simulink library "inp"  (R2021b)
settings: Solver=VariableStepAuto  StartTime=0.0  StopTime=10.0  RelTol=1e-3
undefined symbols (not defined in the file): C_TASK_5MS_S, FALSE, KINP_AcoreReadyToSlp_flg_ovrdflg, KINP_AcoreReadyToSlp_flg_ovrdval, KINP_AllowMovThd_OTA_enum_ovrdflg, KINP_AllowMovThd_OTA_enum_ovrdval, KINP_APSAngleTarget_Deg_ovrdflg, KINP_APSAngleTarget_Deg_ovrdval, KINP_APSDecReq_mps2_ovrdflg, KINP_APSDecReq_mps2_ovrdval, KINP_APSDecReqA_flg_ovrdflg, KINP_APSDecReqA_flg_ovrdval, KINP_APSDFLL_cm_ovrdflg, KINP_APSDFLL_cm_ovrdval, KINP_APSDFLR_cm_ovrdflg, KINP_APSDFLR_cm_ovrdval, KINP_APSDRLL_cm_ovrdflg, KINP_APSDRLL_cm_ovrdval, KINP_APSDRLR_cm_ovrdflg, KINP_APSDRLR_cm_ovrdval, KINP_APSExitCondition_enum_ovrdflg, KINP_APSExitCondition_enum_ovrdval, KINP_APSHWVer_enum_ovrdflg, KINP_APSHWVer_enum_ovrdval, KINP_APSProgressPCT_pct_ovrdflg, KINP_APSProgressPCT_pct_ovrdval, KINP_APSReq_enum_ovrdflg, KINP_APSReq_enum_ovrdval, KINP_APSRQDisplay_enum_ovrdflg, KINP_APSRQDisplay_enum_ovrdval, KINP_APSRqEPASCtrl_flg_ovrdflg, KINP_APSRqEPASCtrl_flg_ovrdval, KINP_APSShiftPosnReq_enum_ovrdval, KINP_APSShiftPosnReq_enum_ovrflg, KINP_APSSpeedCMD_kph_ovrdval, KINP_APSSpeedCMD_kph_ovrflg, KINP_APSStaSystem_enum_ovrdflg, KINP_APSStaSystem_enum_ovrdval, KINP_APSSWVer_enum_ovrdflg, KINP_APSSWVer_enum_ovrdval, KINP_APSVMCReqA_flg_ovrdval, KINP_APSVMCReqA_flg_ovrflg, KINP_APSVRqEPASCtrl_flg_ovrdflg, KINP_APSVRqEPASCtrl_flg_ovrdval, KINP_AuxBattVolmV_mV_ovrdflg, KINP_AuxBattVolmV_mV_ovrdval, KINP_CAASSta_enum_ovrdflg, KINP_CAASSta_enum_ovrdval, KINP_CAASVMCReqA_flg_ovrdval, KINP_CAASVMCReqA_flg_ovrflg, KINP_Chime_enum_ovrdflg, KINP_Chime_enum_ovrdval, KINP_ClearDTCcmd_flg_ovrdflg, KINP_ClearDTCcmd_flg_ovrdval, KINP_EvccAplusPwrUpReq_flg_ovrdflg, KINP_EvccAplusPwrUpReq_flg_ovrdval, KINP_LFID_raw_ovrdval, KINP_LFID_raw_ovrflg, KINP_LRID_raw_ovrdval, KINP_MemOffsetAccX_raw16_ovrdflg ... (+118)
libraries: FVT_lib x595, hcu_lib x1
(part 11 of 27)

== system inp/INP/CAN1/SignalCheck/ESC5 ==
  BHAL_outputs : Inport
  inp_CanValid_bus : Inport  Port=2
  BrkSwSta : FVT_lib/inp/can_signal_template  SystemSampleTime=-1  VariantActivationTime=update diagram  Latency=0  AutoFrameSizeCalculation=off
      link override defval: Value=KINP_BrkSwSta_flg_defval
      link override fftdec: Value=KINP_BrkSwSta_flg_fftdec
      link override fftinc: Value=KINP_BrkSwSta_flg_fftinc
      link override fftlim: Value=KINP_BrkSwSta_flg_fftlim
      link override invalid: Value=KINP_BrkSwSta_flg_invalid
      link override ovrdflg: Value=KINP_BrkSwSta_flg_ovrdflg
      link override ovrdval: Value=KINP_BrkSwSta_flg_ovrdval
      link override setvalid: Value=KINP_BrkSwSta_flg_setvalid
      link override srvcflg: Value=KINP_BrkSwSta_flg_srvcflg
      link override srvcval: Value=KINP_BrkSwSta_flg_srvcval
  BrkSwV : FVT_lib/inp/can_signal_template  SystemSampleTime=-1  VariantActivationTime=update diagram  Latency=0  AutoFrameSizeCalculation=off
      link override defval: Value=KINP_BrkSwV_flg_defval
      link override fftdec: Value=KINP_BrkSwV_flg_fftdec
      link override fftinc: Value=KINP_BrkSwV_flg_fftinc
      link override fftlim: Value=KINP_BrkSwV_flg_fftlim
      link override invalid: Value=KINP_BrkSwV_flg_invalid
      link override ovrdflg: Value=KINP_BrkSwV_flg_ovrdflg
      link override ovrdval: Value=KINP_BrkSwV_flg_ovrdval
      link override setvalid: Value=KINP_BrkSwV_flg_setvalid
      link override srvcflg: Value=KINP_BrkSwV_flg_srvcflg
      link override srvcval: Value=KINP_BrkSwV_flg_srvcval
  ESC5CRC8 : FVT_lib/inp/can_signal_template  SystemSampleTime=-1  VariantActivationTime=update diagram  Latency=0  AutoFrameSizeCalculation=off
      link override defval: Value=KINP_ESC5CRC8_enum_defval
      link override fftdec: Value=KINP_ESC5CRC8_enum_fftdec
      link override fftinc: Value=KINP_ESC5CRC8_enum_fftinc
      link override fftlim: Value=KINP_ESC5CRC8_enum_fftlim
      link override invalid: Value=KINP_ESC5CRC8_enum_invalid
      link override ovrdflg: Value=KINP_ESC5CRC8_enum_ovrdflg
      link override ovrdval: Value=KINP_ESC5CRC8_enum_ovrdval
      link override setvalid: Value=KINP_ESC5CRC8_enum_setvalid
      link override srvcflg: Value=KINP_ESC5CRC8_enum_srvcflg
      link override srvcval: Value=KINP_ESC5CRC8_enum_srvcval
  ESC5CSErr : FVT_lib/inp/can_signal_template  SystemSampleTime=-1  VariantActivationTime=update diagram  Latency=0  AutoFrameSizeCalculation=off
      link override defval: Value=KINP_ESC5CSErr_flg_defval
      link override fftdec: Value=KINP_ESC5CSErr_flg_fftdec
      link override fftinc: Value=KINP_ESC5CSErr_flg_fftinc
      link override fftlim: Value=KINP_ESC5CSErr_flg_fftlim
      link override invalid: Value=KINP_ESC5CSErr_flg_invalid
      link override ovrdflg: Value=KINP_ESC5CSErr_flg_ovrdflg
      link override ovrdval: Value=KINP_ESC5CSErr_flg_ovrdval
      link override setvalid: Value=KINP_ESC5CSErr_flg_setvalid
      link override srvcflg: Value=KINP_ESC5CSErr_flg_srvcflg
      link override srvcval: Value=KINP_ESC5CSErr_flg_srvcval
  ESC5RC : FVT_lib/inp/can_signal_template  SystemSampleTime=-1  VariantActivationTime=update diagram  Latency=0  AutoFrameSizeCalculation=off
      link override defval: Value=KINP_ESC5RC_enum_defval
      link override fftdec: Value=KINP_ESC5RC_enum_fftdec
      link override fftinc: Value=KINP_ESC5RC_enum_fftinc
      link override fftlim: Value=KINP_ESC5RC_enum_fftlim
      link override invalid: Value=KINP_ESC5RC_enum_invalid
      link override ovrdflg: Value=KINP_ESC5RC_enum_ovrdflg
      link override ovrdval: Value=KINP_ESC5RC_enum_ovrdval
      link override setvalid: Value=KINP_ESC5RC_enum_setvalid
      link override srvcflg: Value=KINP_ESC5RC_enum_srvcflg
      link override srvcval: Value=KINP_ESC5RC_enum_srvcval
  ESC5RCErr : FVT_lib/inp/can_signal_template  SystemSampleTime=-1  VariantActivationTime=update diagram  Latency=0  AutoFrameSizeCalculation=off
      link override defval: Value=KINP_ESC5RCErr_flg_defval
      link override fftdec: Value=KINP_ESC5RCErr_flg_fftdec
      link override fftinc: Value=KINP_ESC5RCErr_flg_fftinc
      link override fftlim: Value=KINP_ESC5RCErr_flg_fftlim
      link override invalid: Value=KINP_ESC5RCErr_flg_invalid
      link override ovrdflg: Value=KINP_ESC5RCErr_flg_ovrdflg
      link override ovrdval: Value=KINP_ESC5RCErr_flg_ovrdval
      link override setvalid: Value=KINP_ESC5RCErr_flg_setvalid
      link override srvcflg: Value=KINP_ESC5RCErr_flg_srvcflg
      link override srvcval: Value=KINP_ESC5RCErr_flg_srvcval
  LatAccel : FVT_lib/inp/can_signal_template  SystemSampleTime=-1  VariantActivationTime=update diagram  Latency=0  AutoFrameSizeCalculation=off
      link override defval: Value=KINP_LatAccel_Gps_defval
      link override fftdec: Value=KINP_LatAccel_Gps_fftdec
      link override fftinc: Value=KINP_LatAccel_Gps_fftinc
      link override fftlim: Value=KINP_LatAccel_Gps_fftlim
      link override invalid: Value=KINP_LatAccel_Gps_invalid
      link override ovrdflg: Value=KINP_LatAccel_Gps_ovrdflg
      link override ovrdval: Value=KINP_LatAccel_Gps_ovrdval
      link override setvalid: Value=KINP_LatAccel_Gps_setvalid
      link override srvcflg: Value=KINP_LatAccel_Gps_srvcflg
      link override srvcval: Value=KINP_LatAccel_Gps_srvcval
  LatAccelV : FVT_lib/inp/can_signal_template  SystemSampleTime=-1  VariantActivationTime=update diagram  Latency=0  AutoFrameSizeCalculation=off
      link override defval: Value=KINP_LatAccelV_flg_defval
      link override fftdec: Value=KINP_LatAccelV_flg_fftdec
      link override fftinc: Value=KINP_LatAccelV_flg_fftinc
      link override fftlim: Value=KINP_LatAccelV_flg_fftlim
      link override invalid: Value=KINP_LatAccelV_flg_invalid
      link override ovrdflg: Value=KINP_LatAccelV_flg_ovrdflg
      link override ovrdval: Value=KINP_LatAccelV_flg_ovrdval
      link override setvalid: Value=KINP_LatAccelV_flg_setvalid
      link override srvcflg: Value=KINP_LatAccelV_flg_srvcflg
      link override srvcval: Value=KINP_LatAccelV_flg_srvcval
  LongAccel : FVT_lib/inp/can_signal_template  SystemSampleTime=-1  VariantActivationTime=update diagram  Latency=0  AutoFrameSizeCalculation=off
      link override defval: Value=KINP_LongAccel_Gps_defval
      link override fftdec: Value=KINP_LongAccel_Gps_fftdec
      link override fftinc: Value=KINP_LongAccel_Gps_fftinc
      link override fftlim: Value=KINP_LongAccel_Gps_fftlim
      link override invalid: Value=KINP_LongAccel_Gps_invalid
      link override ovrdflg: Value=KINP_LongAccel_Gps_ovrdflg
      link override ovrdval: Value=KINP_LongAccel_Gps_ovrdval
      link override setvalid: Value=KINP_LongAccel_Gps_setvalid
      link override srvcflg: Value=KINP_LongAccel_Gps_srvcflg
      link override srvcval: Value=KINP_LongAccel_Gps_srvcval
  LongAccelV : FVT_lib/inp/can_signal_template  SystemSampleTime=-1  VariantActivationTime=update diagram  Latency=0  AutoFrameSizeCalculation=off
      link override defval: Value=KINP_LongAccelV_flg_defval
      link override fftdec: Value=KINP_LongAccelV_flg_fftdec
      link override fftinc: Value=KINP_LongAccelV_flg_fftinc
      link override fftlim: Value=KINP_LongAccelV_flg_fftlim
      link override invalid: Value=KINP_LongAccelV_flg_invalid
      link override ovrdflg: Value=KINP_LongAccelV_flg_ovrdflg
      link override ovrdval: Value=KINP_LongAccelV_flg_ovrdval
      link override setvalid: Value=KINP_LongAccelV_flg_setvalid
      link override srvcflg: Value=KINP_LongAccelV_flg_srvcflg
      link override srvcval: Value=KINP_LongAccelV_flg_srvcval
  MCPressure : FVT_lib/inp/can_signal_template  SystemSampleTime=-1  VariantActivationTime=update diagram  Latency=0  AutoFrameSizeCalculation=off
      link override defval: Value=KINP_MCPressure_bar_defval
      link override fftdec: Value=KINP_MCPressure_bar_fftdec
      link override fftinc: Value=KINP_MCPressure_bar_fftinc
      link override fftlim: Value=KINP_MCPressure_bar_fftlim
      link override invalid: Value=KINP_MCPressure_bar_invalid
      link override ovrdflg: Value=KINP_MCPressure_bar_ovrdflg
      link override ovrdval: Value=KINP_MCPressure_bar_ovrdval
      link override setvalid: Value=KINP_MCPressure_bar_setvalid
      link override srvcflg: Value=KINP_MCPressure_bar_srvcflg
      link override srvcval: Value=KINP_MCPressure_bar_srvcval
  MCPressureV : FVT_lib/inp/can_signal_template  SystemSampleTime=-1  VariantActivationTime=update diagram  Latency=0  AutoFrameSizeCalculation=off
      link override defval: Value=KINP_MCPressureV_flg_defval
      link override fftdec: Value=KINP_MCPressureV_flg_fftdec
      link override fftinc: Value=KINP_MCPressureV_flg_fftinc
      link override fftlim: Value=KINP_MCPressureV_flg_fftlim
      link override invalid: Value=KINP_MCPressureV_flg_invalid
      link override ovrdflg: Value=KINP_MCPressureV_flg_ovrdflg
      link override ovrdval: Value=KINP_MCPressureV_flg_ovrdval
      link override setvalid: Value=KINP_MCPressureV_flg_setvalid
      link override srvcflg: Value=KINP_MCPressureV_flg_srvcflg
      link override srvcval: Value=KINP_MCPressureV_flg_srvcval
  Terminator_{1..14} (14 alike) : Terminator
  True_VHAL_BrkSwSta_flg : Constant  Value=TRUE  OutDataTypeStr=boolean
  True_VHAL_BrkSwV_flg : Constant  Value=TRUE  OutDataTypeStr=boolean
  True_VHAL_ESC5CRC8_enum : Constant  Value=TRUE  OutDataTypeStr=boolean
  True_VHAL_ESC5CSErr_flg : Constant  Value=TRUE  OutDataTypeStr=boolean
  True_VHAL_ESC5RCErr_flg : Constant  Value=TRUE  OutDataTypeStr=boolean
  True_VHAL_ESC5RC_enum : Constant  Value=TRUE  OutDataTypeStr=boolean
  True_VHAL_LatAccelV_flg : Constant  Value=TRUE  OutDataTypeStr=boolean
  True_VHAL_LatAccel_Gps : Constant  Value=TRUE  OutDataTypeStr=boolean
  True_VHAL_LongAccelV_flg : Constant  Value=TRUE  OutDataTypeStr=boolean
  True_VHAL_LongAccel_Gps : Constant  Value=TRUE  OutDataTypeStr=boolean
  True_VHAL_MCPressureV_flg : Constant  Value=TRUE  OutDataTypeStr=boolean
  True_VHAL_MCPressure_bar : Constant  Value=TRUE  OutDataTypeStr=boolean
  True_VHAL_YawRateV_flg : Constant  Value=TRUE  OutDataTypeStr=boolean
  True_VHAL_YawRate_degps : Constant  Value=TRUE  OutDataTypeStr=boolean
  YawRate : FVT_lib/inp/can_signal_template  SystemSampleTime=-1  VariantActivationTime=update diagram  Latency=0  AutoFrameSizeCalculation=off
      link override defval: Value=KINP_YawRate_degps_defval
      link override fftdec: Value=KINP_YawRate_degps_fftdec
      link override fftinc: Value=KINP_YawRate_degps_fftinc
      link override fftlim: Value=KINP_YawRate_degps_fftlim
      link override invalid: Value=KINP_YawRate_degps_invalid
      link override ovrdflg: Value=KINP_YawRate_degps_ovrdflg
      link override ovrdval: Value=KINP_YawRate_degps_ovrdval
      link override setvalid: Value=KINP_YawRate_degps_setvalid
      link override srvcflg: Value=KINP_YawRate_degps_srvcflg
      link override srvcval: Value=KINP_YawRate_degps_srvcval
  YawRateV : FVT_lib/inp/can_signal_template  SystemSampleTime=-1  VariantActivationTime=update diagram  Latency=0  AutoFrameSizeCalculation=off
      link override defval: Value=KINP_YawRateV_flg_defval
      link override fftdec: Value=KINP_YawRateV_flg_fftdec
      link override fftinc: Value=KINP_YawRateV_flg_fftinc
      link override fftlim: Value=KINP_YawRateV_flg_fftlim
      link override invalid: Value=KINP_YawRateV_flg_invalid
      link override ovrdflg: Value=KINP_YawRateV_flg_ovrdflg
      link override ovrdval: Value=KINP_YawRateV_flg_ovrdval
      link override setvalid: Value=KINP_YawRateV_flg_setvalid
      link override srvcflg: Value=KINP_YawRateV_flg_srvcflg
      link override srvcval: Value=KINP_YawRateV_flg_srvcval
  slr1_{1..14} (14 alike) : BusSelector  OutputSignals=VINP_CANMsgValidESC5_flg
  slr_VHAL_BrkSwSta_flg : BusSelector  OutputSignals=VHAL_BrkSwSta_flg
  slr_VHAL_BrkSwV_flg : BusSelector  OutputSignals=VHAL_BrkSwV_flg
  slr_VHAL_ESC5CRC8_enum : BusSelector  OutputSignals=VHAL_ESC5CRC8_enum
  slr_VHAL_ESC5CSErr_flg : BusSelector  OutputSignals=VHAL_ESC5CSErr_flg
  slr_VHAL_ESC5RCErr_flg : BusSelector  OutputSignals=VHAL_ESC5RCErr_flg
  slr_VHAL_ESC5RC_enum : BusSelector  OutputSignals=VHAL_ESC5RC_enum
  slr_VHAL_LatAccelV_flg : BusSelector  OutputSignals=VHAL_LatAccelV_flg
  slr_VHAL_LatAccel_Gps : BusSelector  OutputSignals=VHAL_LatAccel_Gps
  slr_VHAL_LongAccelV_flg : BusSelector  OutputSignals=VHAL_LongAccelV_flg
  slr_VHAL_LongAccel_Gps : BusSelector  OutputSignals=VHAL_LongAccel_Gps
  slr_VHAL_MCPressureV_flg : BusSelector  OutputSignals=VHAL_MCPressureV_flg
  slr_VHAL_MCPressure_bar : BusSelector  OutputSignals=VHAL_MCPressure_bar
  slr_VHAL_YawRateV_flg : BusSelector  OutputSignals=VHAL_YawRateV_flg
  slr_VHAL_YawRate_degps : BusSelector  OutputSignals=VHAL_YawRate_degps
  VINP_ESC5CSErr_flg : Outport
  VINP_ESC5RCErr_flg : Outport  Port=2
  VINP_BrkSwSta_flg : Outport  Port=3
  VINP_BrkSwV_flg : Outport  Port=4
  VINP_ESC5CRC8_enum : Outport  Port=5
  VINP_ESC5RC_enum : Outport  Port=6
  VINP_LatAccel_Gps : Outport  Port=7
  VINP_LatAccelV_flg : Outport  Port=8
  VINP_LongAccel_Gps : Outport  Port=9
  VINP_LongAccelV_flg : Outport  Port=10
  VINP_MCPressure_bar : Outport  Port=11
  VINP_MCPressureV_flg : Outport  Port=12
  VINP_YawRate_degps : Outport  Port=13
  VINP_YawRateV_flg : Outport  Port=14
  wires:
  BHAL_outputs/1 -> [BHAL_outputs]
  inp_CanValid_bus/1 -> [inp_CanValid_bus]
  [BHAL_outputs] -> slr_VHAL_ESC5CSErr_flg/1
  slr_VHAL_ESC5CSErr_flg/1 -> ESC5CSErr/1  "<VHAL_ESC5CSErr_flg>"
  True_VHAL_ESC5CSErr_flg/1 -> ESC5CSErr/2
  [inp_CanValid_bus] -> slr1_1/1
  slr1_1/1 -> ESC5CSErr/3  "<VINP_CANMsgValidESC5_flg>"
  ESC5CSErr/1 -> VINP_ESC5CSErr_flg/1  "VINP_ESC5CSErr_flg"
  ESC5CSErr/2 -> Terminator_1/1
  [BHAL_outputs] -> slr_VHAL_ESC5RCErr_flg/1
  slr_VHAL_ESC5RCErr_flg/1 -> ESC5RCErr/1  "<VHAL_ESC5RCErr_flg>"
  True_VHAL_ESC5RCErr_flg/1 -> ESC5RCErr/2
  [inp_CanValid_bus] -> slr1_2/1
  slr1_2/1 -> ESC5RCErr/3  "<VINP_CANMsgValidESC5_flg>"
  ESC5RCErr/1 -> VINP_ESC5RCErr_flg/1  "VINP_ESC5RCErr_flg"
  ESC5RCErr/2 -> Terminator_2/1
  [BHAL_outputs] -> slr_VHAL_BrkSwSta_flg/1
  slr_VHAL_BrkSwSta_flg/1 -> BrkSwSta/1  "<VHAL_BrkSwSta_flg>"
  True_VHAL_BrkSwSta_flg/1 -> BrkSwSta/2
  [inp_CanValid_bus] -> slr1_3/1
  slr1_3/1 -> BrkSwSta/3  "<VINP_CANMsgValidESC5_flg>"
  BrkSwSta/1 -> VINP_BrkSwSta_flg/1  "VINP_BrkSwSta_flg"
  BrkSwSta/2 -> Terminator_3/1
  [BHAL_outputs] -> slr_VHAL_BrkSwV_flg/1
  slr_VHAL_BrkSwV_flg/1 -> BrkSwV/1  "<VHAL_BrkSwV_flg>"
  True_VHAL_BrkSwV_flg/1 -> BrkSwV/2
  [inp_CanValid_bus] -> slr1_4/1
  slr1_4/1 -> BrkSwV/3  "<VINP_CANMsgValidESC5_flg>"
  BrkSwV/1 -> VINP_BrkSwV_flg/1  "VINP_BrkSwV_flg"
  BrkSwV/2 -> Terminator_4/1
  [BHAL_outputs] -> slr_VHAL_ESC5CRC8_enum/1
  slr_VHAL_ESC5CRC8_enum/1 -> ESC5CRC8/1  "<VHAL_ESC5CRC8_enum>"
  True_VHAL_ESC5CRC8_enum/1 -> ESC5CRC8/2
  [inp_CanValid_bus] -> slr1_5/1
  slr1_5/1 -> ESC5CRC8/3  "<VINP_CANMsgValidESC5_flg>"
  ESC5CRC8/1 -> VINP_ESC5CRC8_enum/1  "VINP_ESC5CRC8_enum"
  ESC5CRC8/2 -> Terminator_5/1
  [BHAL_outputs] -> slr_VHAL_ESC5RC_enum/1
  slr_VHAL_ESC5RC_enum/1 -> ESC5RC/1  "<VHAL_ESC5RC_enum>"
  True_VHAL_ESC5RC_enum/1 -> ESC5RC/2
  [inp_CanValid_bus] -> slr1_6/1
  slr1_6/1 -> ESC5RC/3  "<VINP_CANMsgValidESC5_flg>"
  ESC5RC/1 -> VINP_ESC5RC_enum/1  "VINP_ESC5RC_enum"
  ESC5RC/2 -> Terminator_6/1
  [BHAL_outputs] -> slr_VHAL_LatAccel_Gps/1
  slr_VHAL_LatAccel_Gps/1 -> LatAccel/1  "<VHAL_LatAccel_Gps>"
  True_VHAL_LatAccel_Gps/1 -> LatAccel/2
  [inp_CanValid_bus] -> slr1_7/1
  slr1_7/1 -> LatAccel/3  "<VINP_CANMsgValidESC5_flg>"
  LatAccel/1 -> VINP_LatAccel_Gps/1  "VINP_LatAccel_Gps"
  LatAccel/2 -> Terminator_7/1
  [BHAL_outputs] -> slr_VHAL_LatAccelV_flg/1
  slr_VHAL_LatAccelV_flg/1 -> LatAccelV/1  "<VHAL_LatAccelV_flg>"
  True_VHAL_LatAccelV_flg/1 -> LatAccelV/2
  [inp_CanValid_bus] -> slr1_8/1
  slr1_8/1 -> LatAccelV/3  "<VINP_CANMsgValidESC5_flg>"
  LatAccelV/1 -> VINP_LatAccelV_flg/1  "VINP_LatAccelV_flg"
  LatAccelV/2 -> Terminator_8/1
  [BHAL_outputs] -> slr_VHAL_LongAccel_Gps/1
  slr_VHAL_LongAccel_Gps/1 -> LongAccel/1  "<VHAL_LongAccel_Gps>"
  True_VHAL_LongAccel_Gps/1 -> LongAccel/2
  [inp_CanValid_bus] -> slr1_9/1
  slr1_9/1 -> LongAccel/3  "<VINP_CANMsgValidESC5_flg>"
  LongAccel/1 -> VINP_LongAccel_Gps/1  "VINP_LongAccel_Gps"
  LongAccel/2 -> Terminator_9/1
  [BHAL_outputs] -> slr_VHAL_LongAccelV_flg/1
  slr_VHAL_LongAccelV_flg/1 -> LongAccelV/1  "<VHAL_LongAccelV_flg>"
  True_VHAL_LongAccelV_flg/1 -> LongAccelV/2
  [inp_CanValid_bus] -> slr1_10/1
  slr1_10/1 -> LongAccelV/3  "<VINP_CANMsgValidESC5_flg>"
  LongAccelV/1 -> VINP_LongAccelV_flg/1  "VINP_LongAccelV_flg"
  LongAccelV/2 -> Terminator_10/1
  [BHAL_outputs] -> slr_VHAL_MCPressure_bar/1
  slr_VHAL_MCPressure_bar/1 -> MCPressure/1  "<VHAL_MCPressure_bar>"
  True_VHAL_MCPressure_bar/1 -> MCPressure/2
  [inp_CanValid_bus] -> slr1_11/1
  slr1_11/1 -> MCPressure/3  "<VINP_CANMsgValidESC5_flg>"
  MCPressure/1 -> VINP_MCPressure_bar/1  "VINP_MCPressure_bar"
  MCPressure/2 -> Terminator_11/1
  [BHAL_outputs] -> slr_VHAL_MCPressureV_flg/1
  slr_VHAL_MCPressureV_flg/1 -> MCPressureV/1  "<VHAL_MCPressureV_flg>"
  True_VHAL_MCPressureV_flg/1 -> MCPressureV/2
  [inp_CanValid_bus] -> slr1_12/1
  slr1_12/1 -> MCPressureV/3  "<VINP_CANMsgValidESC5_flg>"
  MCPressureV/1 -> VINP_MCPressureV_flg/1  "VINP_MCPressureV_flg"
  MCPressureV/2 -> Terminator_12/1
  [BHAL_outputs] -> slr_VHAL_YawRate_degps/1
  slr_VHAL_YawRate_degps/1 -> YawRate/1  "<VHAL_YawRate_degps>"
  True_VHAL_YawRate_degps/1 -> YawRate/2
  [inp_CanValid_bus] -> slr1_13/1
  slr1_13/1 -> YawRate/3  "<VINP_CANMsgValidESC5_flg>"
  YawRate/1 -> VINP_YawRate_degps/1  "VINP_YawRate_degps"
  YawRate/2 -> Terminator_13/1
  [BHAL_outputs] -> slr_VHAL_YawRateV_flg/1
  slr_VHAL_YawRateV_flg/1 -> YawRateV/1  "<VHAL_YawRateV_flg>"
  True_VHAL_YawRateV_flg/1 -> YawRateV/2
  [inp_CanValid_bus] -> slr1_14/1
  slr1_14/1 -> YawRateV/3  "<VINP_CANMsgValidESC5_flg>"
  YawRateV/1 -> VINP_YawRateV_flg/1  "VINP_YawRateV_flg"
  YawRateV/2 -> Terminator_14/1

== system inp/INP/CAN1/SignalCheck/ESC6 ==
  BHAL_outputs : Inport
  inp_CanValid_bus : Inport  Port=2
  ActBrkLampSta : FVT_lib/inp/can_signal_template  SystemSampleTime=-1  VariantActivationTime=update diagram  Latency=0  AutoFrameSizeCalculation=off
      link override defval: Value=KINP_ActBrkLampSta_flg_defval
      link override fftdec: Value=KINP_ActBrkLampSta_flg_fftdec
      link override fftinc: Value=KINP_ActBrkLampSta_flg_fftinc
      link override fftlim: Value=KINP_ActBrkLampSta_flg_fftlim
      link override invalid: Value=KINP_ActBrkLampSta_flg_invalid
      link override ovrdflg: Value=KINP_ActBrkLampSta_flg_ovrdflg
      link override ovrdval: Value=KINP_ActBrkLampSta_flg_ovrdval
      link override setvalid: Value=KINP_ActBrkLampSta_flg_setvalid
      link override srvcflg: Value=KINP_ActBrkLampSta_flg_srvcflg
      link override srvcval: Value=KINP_ActBrkLampSta_flg_srvcval
  ESCADASSta : FVT_lib/inp/can_signal_template  SystemSampleTime=-1  VariantActivationTime=update diagram  Latency=0  AutoFrameSizeCalculation=off
      link override defval: Value=KINP_ESCADASSta_enum_defval
      link override fftdec: Value=KINP_ESCADASSta_enum_fftdec
      link override fftinc: Value=KINP_ESCADASSta_enum_fftinc
      link override fftlim: Value=KINP_ESCADASSta_enum_fftlim
      link override invalid: Value=KINP_ESCADASSta_enum_invalid
      link override ovrdflg: Value=KINP_ESCADASSta_enum_ovrdflg
      link override ovrdval: Value=KINP_ESCADASSta_enum_ovrdval
      link override setvalid: Value=KINP_ESCADASSta_enum_setvalid
      link override srvcflg: Value=KINP_ESCADASSta_enum_srvcflg
      link override srvcval: Value=KINP_ESCADASSta_enum_srvcval
  ESCAPSSta : FVT_lib/inp/can_signal_template  SystemSampleTime=-1  VariantActivationTime=update diagram  Latency=0  AutoFrameSizeCalculation=off
      link override defval: Value=KINP_ESCAPSSta_enum_defval
      link override fftdec: Value=KINP_ESCAPSSta_enum_fftdec
      link override fftinc: Value=KINP_ESCAPSSta_enum_fftinc
      link override fftlim: Value=KINP_ESCAPSSta_enum_fftlim
      link override invalid: Value=KINP_ESCAPSSta_enum_invalid
      link override ovrdflg: Value=KINP_ESCAPSSta_enum_ovrdflg
      link override ovrdval: Value=KINP_ESCAPSSta_enum_ovrdval
      link override setvalid: Value=KINP_ESCAPSSta_enum_setvalid
      link override srvcflg: Value=KINP_ESCAPSSta_enum_srvcflg
      link override srvcval: Value=KINP_ESCAPSSta_enum_srvcval
  ESCStandstill : FVT_lib/inp/can_signal_template  SystemSampleTime=-1  VariantActivationTime=update diagram  Latency=0  AutoFrameSizeCalculation=off
      link override defval: Value=KINP_ESCStandstill_flg_defval
      link override fftdec: Value=KINP_ESCStandstill_flg_fftdec
      link override fftinc: Value=KINP_ESCStandstill_flg_fftinc
      link override fftlim: Value=KINP_ESCStandstill_flg_fftlim
      link override invalid: Value=KINP_ESCStandstill_flg_invalid
      link override ovrdflg: Value=KINP_ESCStandstill_flg_ovrdflg
      link override ovrdval: Value=KINP_ESCStandstill_flg_ovrdval
      link override setvalid: Value=KINP_ESCStandstill_flg_setvalid
      link override srvcflg: Value=KINP_ESCStandstill_flg_srvcflg
      link override srvcval: Value=KINP_ESCStandstill_flg_srvcval
  Terminator_{1..4} (4 alike) : Terminator
  True_VHAL_ActBrkLampSta_flg : Constant  Value=TRUE  OutDataTypeStr=boolean
  True_VHAL_ESCADASSta_enum : Constant  Value=TRUE  OutDataTypeStr=boolean
  True_VHAL_ESCAPSSta_enum : Constant  Value=TRUE  OutDataTypeStr=boolean
  True_VHAL_ESCStandstill_flg : Constant  Value=TRUE  OutDataTypeStr=boolean
  slr1_{1..4} (4 alike) : BusSelector  OutputSignals=VINP_CANMsgValidESC6_flg
  slr_VHAL_ActBrkLampSta_flg : BusSelector  OutputSignals=VHAL_ActBrkLampSta_flg
  slr_VHAL_ESCADASSta_enum : BusSelector  OutputSignals=VHAL_ESCADASSta_enum
  slr_VHAL_ESCAPSSta_enum : BusSelector  OutputSignals=VHAL_ESCAPSSta_enum
  slr_VHAL_ESCStandstill_flg : BusSelector  OutputSignals=VHAL_ESCStandstill_flg
  VINP_ActBrkLampSta_flg : Outport
  VINP_ESCADASSta_enum : Outport  Port=2
  VINP_ESCAPSSta_enum : Outport  Port=3
  VINP_ESCStandstill_flg : Outport  Port=4
  wires:
  BHAL_outputs/1 -> [BHAL_outputs]
  inp_CanValid_bus/1 -> [inp_CanValid_bus]
  [BHAL_outputs] -> slr_VHAL_ActBrkLampSta_flg/1
  slr_VHAL_ActBrkLampSta_flg/1 -> ActBrkLampSta/1  "<VHAL_ActBrkLampSta_flg>"
  True_VHAL_ActBrkLampSta_flg/1 -> ActBrkLampSta/2
  [inp_CanValid_bus] -> slr1_1/1
  slr1_1/1 -> ActBrkLampSta/3  "<VINP_CANMsgValidESC6_flg>"
  ActBrkLampSta/1 -> VINP_ActBrkLampSta_flg/1  "VINP_ActBrkLampSta_flg"
  ActBrkLampSta/2 -> Terminator_1/1
  [BHAL_outputs] -> slr_VHAL_ESCADASSta_enum/1
  slr_VHAL_ESCADASSta_enum/1 -> ESCADASSta/1  "<VHAL_ESCADASSta_enum>"
  True_VHAL_ESCADASSta_enum/1 -> ESCADASSta/2
  [inp_CanValid_bus] -> slr1_2/1
  slr1_2/1 -> ESCADASSta/3  "<VINP_CANMsgValidESC6_flg>"
  ESCADASSta/1 -> VINP_ESCADASSta_enum/1  "VINP_ESCADASSta_enum"
  ESCADASSta/2 -> Terminator_2/1
  [BHAL_outputs] -> slr_VHAL_ESCAPSSta_enum/1
  slr_VHAL_ESCAPSSta_enum/1 -> ESCAPSSta/1  "<VHAL_ESCAPSSta_enum>"
  True_VHAL_ESCAPSSta_enum/1 -> ESCAPSSta/2
  [inp_CanValid_bus] -> slr1_3/1
  slr1_3/1 -> ESCAPSSta/3  "<VINP_CANMsgValidESC6_flg>"
  ESCAPSSta/1 -> VINP_ESCAPSSta_enum/1  "VINP_ESCAPSSta_enum"
  ESCAPSSta/2 -> Terminator_3/1
  [BHAL_outputs] -> slr_VHAL_ESCStandstill_flg/1
  slr_VHAL_ESCStandstill_flg/1 -> ESCStandstill/1  "<VHAL_ESCStandstill_flg>"
  True_VHAL_ESCStandstill_flg/1 -> ESCStandstill/2
  [inp_CanValid_bus] -> slr1_4/1
  slr1_4/1 -> ESCStandstill/3  "<VINP_CANMsgValidESC6_flg>"
  ESCStandstill/1 -> VINP_ESCStandstill_flg/1  "VINP_ESCStandstill_flg"
  ESCStandstill/2 -> Terminator_4/1

== system inp/INP/CAN1/SignalCheck/ESC7 ==
  BHAL_outputs : Inport
  inp_CanValid_bus : Inport  Port=2
  BrkPedalPos : FVT_lib/inp/can_signal_template  SystemSampleTime=-1  VariantActivationTime=update diagram  Latency=0  AutoFrameSizeCalculation=off
      link override defval: Value=KINP_BrkPedalPos_pct_defval
      link override fftdec: Value=KINP_BrkPedalPos_pct_fftdec
      link override fftinc: Value=KINP_BrkPedalPos_pct_fftinc
      link override fftlim: Value=KINP_BrkPedalPos_pct_fftlim
      link override invalid: Value=KINP_BrkPedalPos_pct_invalid
      link override ovrdflg: Value=KINP_BrkPedalPos_pct_ovrdflg
      link override ovrdval: Value=KINP_BrkPedalPos_pct_ovrdval
      link override setvalid: Value=KINP_BrkPedalPos_pct_setvalid
      link override srvcflg: Value=KINP_BrkPedalPos_pct_srvcflg
      link override srvcval: Value=KINP_BrkPedalPos_pct_srvcval
  BrkPedalPosSta : FVT_lib/inp/can_signal_template  SystemSampleTime=-1  VariantActivationTime=update diagram  Latency=0  AutoFrameSizeCalculation=off
      link override defval: Value=KINP_BrkPedalPosSta_flg_defval
      link override fftdec: Value=KINP_BrkPedalPosSta_flg_fftdec
      link override fftinc: Value=KINP_BrkPedalPosSta_flg_fftinc
      link override fftlim: Value=KINP_BrkPedalPosSta_flg_fftlim
      link override invalid: Value=KINP_BrkPedalPosSta_flg_invalid
      link override ovrdflg: Value=KINP_BrkPedalPosSta_flg_ovrdflg
      link override ovrdval: Value=KINP_BrkPedalPosSta_flg_ovrdval
      link override setvalid: Value=KINP_BrkPedalPosSta_flg_setvalid
      link override srvcflg: Value=KINP_BrkPedalPosSta_flg_srvcflg
      link override srvcval: Value=KINP_BrkPedalPosSta_flg_srvcval
  ESC7CS : FVT_lib/inp/can_signal_template  SystemSampleTime=-1  VariantActivationTime=update diagram  Latency=0  AutoFrameSizeCalculation=off
      link override defval: Value=KINP_ESC7CS_enum_defval
      link override fftdec: Value=KINP_ESC7CS_enum_fftdec
      link override fftinc: Value=KINP_ESC7CS_enum_fftinc
      link override fftlim: Value=KINP_ESC7CS_enum_fftlim
      link override invalid: Value=KINP_ESC7CS_enum_invalid
      link override ovrdflg: Value=KINP_ESC7CS_enum_ovrdflg
      link override ovrdval: Value=KINP_ESC7CS_enum_ovrdval
      link override setvalid: Value=KINP_ESC7CS_enum_setvalid
      link override srvcflg: Value=KINP_ESC7CS_enum_srvcflg
      link override srvcval: Value=KINP_ESC7CS_enum_srvcval
  ESC7CSErr : FVT_lib/inp/can_signal_template  SystemSampleTime=-1  VariantActivationTime=update diagram  Latency=0  AutoFrameSizeCalculation=off
      link override defval: Value=KINP_ESC7CSErr_flg_defval
      link override fftdec: Value=KINP_ESC7CSErr_flg_fftdec
      link override fftinc: Value=KINP_ESC7CSErr_flg_fftinc
      link override fftlim: Value=KINP_ESC7CSErr_flg_fftlim
      link override invalid: Value=KINP_ESC7CSErr_flg_invalid
      link override ovrdflg: Value=KINP_ESC7CSErr_flg_ovrdflg
      link override ovrdval: Value=KINP_ESC7CSErr_flg_ovrdval
      link override setvalid: Value=KINP_ESC7CSErr_flg_setvalid
      link override srvcflg: Value=KINP_ESC7CSErr_flg_srvcflg
      link override srvcval: Value=KINP_ESC7CSErr_flg_srvcval
  ESC7RC : FVT_lib/inp/can_signal_template  SystemSampleTime=-1  VariantActivationTime=update diagram  Latency=0  AutoFrameSizeCalculation=off
      link override defval: Value=KINP_ESC7RC_enum_defval
      link override fftdec: Value=KINP_ESC7RC_enum_fftdec
      link override fftinc: Value=KINP_ESC7RC_enum_fftinc
      link override fftlim: Value=KINP_ESC7RC_enum_fftlim
      link override invalid: Value=KINP_ESC7RC_enum_invalid
      link override ovrdflg: Value=KINP_ESC7RC_enum_ovrdflg
      link override ovrdval: Value=KINP_ESC7RC_enum_ovrdval
      link override setvalid: Value=KINP_ESC7RC_enum_setvalid
      link override srvcflg: Value=KINP_ESC7RC_enum_srvcflg
      link override srvcval: Value=KINP_ESC7RC_enum_srvcval
  ESC7RCErr : FVT_lib/inp/can_signal_template  SystemSampleTime=-1  VariantActivationTime=update diagram  Latency=0  AutoFrameSizeCalculation=off
      link override defval: Value=KINP_ESC7RCErr_flg_defval
      link override fftdec: Value=KINP_ESC7RCErr_flg_fftdec
      link override fftinc: Value=KINP_ESC7RCErr_flg_fftinc
      link override fftlim: Value=KINP_ESC7RCErr_flg_fftlim
      link override invalid: Value=KINP_ESC7RCErr_flg_invalid
      link override ovrdflg: Value=KINP_ESC7RCErr_flg_ovrdflg
      link override ovrdval: Value=KINP_ESC7RCErr_flg_ovrdval
      link override setvalid: Value=KINP_ESC7RCErr_flg_setvalid
      link override srvcflg: Value=KINP_ESC7RCErr_flg_srvcflg
      link override srvcval: Value=KINP_ESC7RCErr_flg_srvcval
  FrRBCActive : FVT_lib/inp/can_signal_template  SystemSampleTime=-1  VariantActivationTime=update diagram  Latency=0  AutoFrameSizeCalculation=off
      link override defval: Value=KINP_FrRBCActive_flg_defval
      link override fftdec: Value=KINP_FrRBCActive_flg_fftdec
      link override fftinc: Value=KINP_FrRBCActive_flg_fftinc
      link override fftlim: Value=KINP_FrRBCActive_flg_fftlim
      link override invalid: Value=KINP_FrRBCActive_flg_invalid
      link override ovrdflg: Value=KINP_FrRBCActive_flg_ovrdflg
      link override ovrdval: Value=KINP_FrRBCActive_flg_ovrdval
      link override setvalid: Value=KINP_FrRBCActive_flg_setvalid
      link override srvcflg: Value=KINP_FrRBCActive_flg_srvcflg
      link override srvcval: Value=KINP_FrRBCActive_flg_srvcval
  FrntAxlTrqReqBrk : FVT_lib/inp/can_signal_template  SystemSampleTime=-1  VariantActivationTime=update diagram  Latency=0  AutoFrameSizeCalculation=off
      link override defval: Value=KINP_FrntAxlTrqReqBrk_Nm_defval
      link override fftdec: Value=KINP_FrntAxlTrqReqBrk_Nm_fftdec
      link override fftinc: Value=KINP_FrntAxlTrqReqBrk_Nm_fftinc
      link override fftlim: Value=KINP_FrntAxlTrqReqBrk_Nm_fftlim
      link override invalid: Value=KINP_FrntAxlTrqReqBrk_Nm_invalid
      link override ovrdflg: Value=KINP_FrntAxlTrqReqBrk_Nm_ovrdflg
      link override ovrdval: Value=KINP_FrntAxlTrqReqBrk_Nm_ovrdval
      link override setvalid: Value=KINP_FrntAxlTrqReqBrk_Nm_setvalid
      link override srvcflg: Value=KINP_FrntAxlTrqReqBrk_Nm_srvcflg
      link override srvcval: Value=KINP_FrntAxlTrqReqBrk_Nm_srvcval
  RDCActive : FVT_lib/inp/can_signal_template  SystemSampleTime=-1  VariantActivationTime=update diagram  Latency=0  AutoFrameSizeCalculation=off
      link override defval: Value=KINP_RDCActive_enum_defval
      link override fftdec: Value=KINP_RDCActive_enum_fftdec
      link override fftinc: Value=KINP_RDCActive_enum_fftinc
      link override fftlim: Value=KINP_RDCActive_enum_fftlim
      link override invalid: Value=KINP_RDCActive_enum_invalid
      link override ovrdflg: Value=KINP_RDCActive_enum_ovrdflg
      link override ovrdval: Value=KINP_RDCActive_enum_ovrdval
      link override setvalid: Value=KINP_RDCActive_enum_setvalid
      link override srvcflg: Value=KINP_RDCActive_enum_srvcflg
      link override srvcval: Value=KINP_RDCActive_enum_srvcval
  RearAxlTrqReqBrk : FVT_lib/inp/can_signal_template  SystemSampleTime=-1  VariantActivationTime=update diagram  Latency=0  AutoFrameSizeCalculation=off
      link override defval: Value=KINP_RearAxlTrqReqBrk_Nm_defval
      link override fftdec: Value=KINP_RearAxlTrqReqBrk_Nm_fftdec
      link override fftinc: Value=KINP_RearAxlTrqReqBrk_Nm_fftinc
      link override fftlim: Value=KINP_RearAxlTrqReqBrk_Nm_fftlim
      link override invalid: Value=KINP_RearAxlTrqReqBrk_Nm_invalid
      link override ovrdflg: Value=KINP_RearAxlTrqReqBrk_Nm_ovrdflg
      link override ovrdval: Value=KINP_RearAxlTrqReqBrk_Nm_ovrdval
      link override setvalid: Value=KINP_RearAxlTrqReqBrk_Nm_setvalid
      link override srvcflg: Value=KINP_RearAxlTrqReqBrk_Nm_srvcflg
      link override srvcval: Value=KINP_RearAxlTrqReqBrk_Nm_srvcval
  RrRBCActive : FVT_lib/inp/can_signal_template  SystemSampleTime=-1  VariantActivationTime=update diagram  Latency=0  AutoFrameSizeCalculation=off
      link override defval: Value=KINP_RrRBCActive_flg_defval
      link override fftdec: Value=KINP_RrRBCActive_flg_fftdec
      link override fftinc: Value=KINP_RrRBCActive_flg_fftinc
      link override fftlim: Value=KINP_RrRBCActive_flg_fftlim
      link override invalid: Value=KINP_RrRBCActive_flg_invalid
      link override ovrdflg: Value=KINP_RrRBCActive_flg_ovrdflg
      link override ovrdval: Value=KINP_RrRBCActive_flg_ovrdval
      link override setvalid: Value=KINP_RrRBCActive_flg_setvalid
      link override srvcflg: Value=KINP_RrRBCActive_flg_srvcflg
      link override srvcval: Value=KINP_RrRBCActive_flg_srvcval
  Terminator_{1..11} (11 alike) : Terminator
  True_VHAL_BrkPedalPosSta_flg : Constant  Value=TRUE  OutDataTypeStr=boolean
  True_VHAL_BrkPedalPos_pct : Constant  Value=TRUE  OutDataTypeStr=boolean
  True_VHAL_ESC7CSErr_flg : Constant  Value=TRUE  OutDataTypeStr=boolean
  True_VHAL_ESC7CS_enum : Constant  Value=TRUE  OutDataTypeStr=boolean
  True_VHAL_ESC7RCErr_flg : Constant  Value=TRUE  OutDataTypeStr=boolean
  True_VHAL_ESC7RC_enum : Constant  Value=TRUE  OutDataTypeStr=boolean
  True_VHAL_FrRBCActive_flg : Constant  Value=TRUE  OutDataTypeStr=boolean
  True_VHAL_FrntAxlTrqReqBrk_Nm : Constant  Value=TRUE  OutDataTypeStr=boolean
  True_VHAL_RDCActive_enum : Constant  Value=TRUE  OutDataTypeStr=boolean
  True_VHAL_RearAxlTrqReqBrk_Nm : Constant  Value=TRUE  OutDataTypeStr=boolean
  True_VHAL_RrRBCActive_flg : Constant  Value=TRUE  OutDataTypeStr=boolean
  slr1_{1..11} (11 alike) : BusSelector  OutputSignals=VINP_CANMsgValidESC7_flg
  slr_VHAL_BrkPedalPosSta_flg : BusSelector  OutputSignals=VHAL_BrkPedalPosSta_flg
  slr_VHAL_BrkPedalPos_pct : BusSelector  OutputSignals=VHAL_BrkPedalPos_pct
  slr_VHAL_ESC7CSErr_flg : BusSelector  OutputSignals=VHAL_ESC7CSErr_flg
  slr_VHAL_ESC7CS_enum : BusSelector  OutputSignals=VHAL_ESC7CS_enum
  slr_VHAL_ESC7RCErr_flg : BusSelector  OutputSignals=VHAL_ESC7RCErr_flg
  slr_VHAL_ESC7RC_enum : BusSelector  OutputSignals=VHAL_ESC7RC_enum
  slr_VHAL_FrRBCActive_flg : BusSelector  OutputSignals=VHAL_FrRBCActive_flg
  slr_VHAL_FrntAxlTrqReqBrk_Nm : BusSelector  OutputSignals=VHAL_FrntAxlTrqReqBrk_Nm
  slr_VHAL_RDCActive_enum : BusSelector  OutputSignals=VHAL_RDCActive_enum
  slr_VHAL_RearAxlTrqReqBrk_Nm : BusSelector  OutputSignals=VHAL_RearAxlTrqReqBrk_Nm
  slr_VHAL_RrRBCActive_flg : BusSelector  OutputSignals=VHAL_RrRBCActive_flg
  VINP_ESC7CSErr_flg : Outport
  VINP_ESC7RCErr_flg : Outport  Port=2
  VINP_BrkPedalPos_pct : Outport  Port=3
  VINP_BrkPedalPosSta_flg : Outport  Port=4
  VINP_ESC7CS_enum : Outport  Port=5
  VINP_ESC7RC_enum : Outport  Port=6
  VINP_FrRBCActive_flg : Outport  Port=7
  VINP_FrntAxlTrqReqBrk_Nm : Outport  Port=8
  VINP_RDCActive_enum : Outport  Port=9
  VINP_RearAxlTrqReqBrk_Nm : Outport  Port=10
  VINP_RrRBCActive_flg : Outport  Port=11
  wires:
  BHAL_outputs/1 -> [BHAL_outputs]
  inp_CanValid_bus/1 -> [inp_CanValid_bus]
  [BHAL_outputs] -> slr_VHAL_ESC7CSErr_flg/1
  slr_VHAL_ESC7CSErr_flg/1 -> ESC7CSErr/1  "<VHAL_ESC7CSErr_flg>"
  True_VHAL_ESC7CSErr_flg/1 -> ESC7CSErr/2
  [inp_CanValid_bus] -> slr1_1/1
  slr1_1/1 -> ESC7CSErr/3  "<VINP_CANMsgValidESC7_flg>"
  ESC7CSErr/1 -> VINP_ESC7CSErr_flg/1  "VINP_ESC7CSErr_flg"
  ESC7CSErr/2 -> Terminator_1/1
  [BHAL_outputs] -> slr_VHAL_ESC7RCErr_flg/1
  slr_VHAL_ESC7RCErr_flg/1 -> ESC7RCErr/1  "<VHAL_ESC7RCErr_flg>"
  True_VHAL_ESC7RCErr_flg/1 -> ESC7RCErr/2
  [inp_CanValid_bus] -> slr1_2/1
  slr1_2/1 -> ESC7RCErr/3  "<VINP_CANMsgValidESC7_flg>"
  ESC7RCErr/1 -> VINP_ESC7RCErr_flg/1  "VINP_ESC7RCErr_flg"
  ESC7RCErr/2 -> Terminator_2/1
  [BHAL_outputs] -> slr_VHAL_BrkPedalPos_pct/1
  slr_VHAL_BrkPedalPos_pct/1 -> BrkPedalPos/1  "<VHAL_BrkPedalPos_pct>"
  True_VHAL_BrkPedalPos_pct/1 -> BrkPedalPos/2
  [inp_CanValid_bus] -> slr1_3/1
  slr1_3/1 -> BrkPedalPos/3  "<VINP_CANMsgValidESC7_flg>"
  BrkPedalPos/1 -> VINP_BrkPedalPos_pct/1  "VINP_BrkPedalPos_pct"
  BrkPedalPos/2 -> Terminator_3/1
  [BHAL_outputs] -> slr_VHAL_BrkPedalPosSta_flg/1
  slr_VHAL_BrkPedalPosSta_flg/1 -> BrkPedalPosSta/1  "<VHAL_BrkPedalPosSta_flg>"
  True_VHAL_BrkPedalPosSta_flg/1 -> BrkPedalPosSta/2
  [inp_CanValid_bus] -> slr1_4/1
  slr1_4/1 -> BrkPedalPosSta/3  "<VINP_CANMsgValidESC7_flg>"
  BrkPedalPosSta/1 -> VINP_BrkPedalPosSta_flg/1  "VINP_BrkPedalPosSta_flg"
  BrkPedalPosSta/2 -> Terminator_4/1
  [BHAL_outputs] -> slr_VHAL_ESC7CS_enum/1
  slr_VHAL_ESC7CS_enum/1 -> ESC7CS/1  "<VHAL_ESC7CS_enum>"
  True_VHAL_ESC7CS_enum/1 -> ESC7CS/2
  [inp_CanValid_bus] -> slr1_5/1
  slr1_5/1 -> ESC7CS/3  "<VINP_CANMsgValidESC7_flg>"
  ESC7CS/1 -> VINP_ESC7CS_enum/1  "VINP_ESC7CS_enum"
  ESC7CS/2 -> Terminator_5/1
  [BHAL_outputs] -> slr_VHAL_ESC7RC_enum/1
  slr_VHAL_ESC7RC_enum/1 -> ESC7RC/1  "<VHAL_ESC7RC_enum>"
  True_VHAL_ESC7RC_enum/1 -> ESC7RC/2
  [inp_CanValid_bus] -> slr1_6/1
  slr1_6/1 -> ESC7RC/3  "<VINP_CANMsgValidESC7_flg>"
  ESC7RC/1 -> VINP_ESC7RC_enum/1  "VINP_ESC7RC_enum"
  ESC7RC/2 -> Terminator_6/1
  [BHAL_outputs] -> slr_VHAL_FrRBCActive_flg/1
  slr_VHAL_FrRBCActive_flg/1 -> FrRBCActive/1  "<VHAL_FrRBCActive_flg>"
  True_VHAL_FrRBCActive_flg/1 -> FrRBCActive/2
  [inp_CanValid_bus] -> slr1_7/1
  slr1_7/1 -> FrRBCActive/3  "<VINP_CANMsgValidESC7_flg>"
  FrRBCActive/1 -> VINP_FrRBCActive_flg/1  "VINP_FrRBCActive_flg"
  FrRBCActive/2 -> Terminator_7/1
  [BHAL_outputs] -> slr_VHAL_FrntAxlTrqReqBrk_Nm/1
  slr_VHAL_FrntAxlTrqReqBrk_Nm/1 -> FrntAxlTrqReqBrk/1  "<VHAL_FrntAxlTrqReqBrk_Nm>"
  True_VHAL_FrntAxlTrqReqBrk_Nm/1 -> FrntAxlTrqReqBrk/2
  [inp_CanValid_bus] -> slr1_8/1
  slr1_8/1 -> FrntAxlTrqReqBrk/3  "<VINP_CANMsgValidESC7_flg>"
  FrntAxlTrqReqBrk/1 -> VINP_FrntAxlTrqReqBrk_Nm/1  "VINP_FrntAxlTrqReqBrk_Nm"
  FrntAxlTrqReqBrk/2 -> Terminator_8/1
  [BHAL_outputs] -> slr_VHAL_RDCActive_enum/1
  slr_VHAL_RDCActive_enum/1 -> RDCActive/1  "<VHAL_RDCActive_enum>"
  True_VHAL_RDCActive_enum/1 -> RDCActive/2
  [inp_CanValid_bus] -> slr1_9/1
  slr1_9/1 -> RDCActive/3  "<VINP_CANMsgValidESC7_flg>"
  RDCActive/1 -> VINP_RDCActive_enum/1  "VINP_RDCActive_enum"
  RDCActive/2 -> Terminator_9/1
  [BHAL_outputs] -> slr_VHAL_RearAxlTrqReqBrk_Nm/1
  slr_VHAL_RearAxlTrqReqBrk_Nm/1 -> RearAxlTrqReqBrk/1  "<VHAL_RearAxlTrqReqBrk_Nm>"
  True_VHAL_RearAxlTrqReqBrk_Nm/1 -> RearAxlTrqReqBrk/2
  [inp_CanValid_bus] -> slr1_10/1
  slr1_10/1 -> RearAxlTrqReqBrk/3  "<VINP_CANMsgValidESC7_flg>"
  RearAxlTrqReqBrk/1 -> VINP_RearAxlTrqReqBrk_Nm/1  "VINP_RearAxlTrqReqBrk_Nm"
  RearAxlTrqReqBrk/2 -> Terminator_10/1
  [BHAL_outputs] -> slr_VHAL_RrRBCActive_flg/1
  slr_VHAL_RrRBCActive_flg/1 -> RrRBCActive/1  "<VHAL_RrRBCActive_flg>"
  True_VHAL_RrRBCActive_flg/1 -> RrRBCActive/2
  [inp_CanValid_bus] -> slr1_11/1
  slr1_11/1 -> RrRBCActive/3  "<VINP_CANMsgValidESC7_flg>"
  RrRBCActive/1 -> VINP_RrRBCActive_flg/1  "VINP_RrRBCActive_flg"
  RrRBCActive/2 -> Terminator_11/1

== system inp/INP/CAN1/SignalCheck/FCM2 ==
  BHAL_outputs : Inport
  inp_CanValid_bus : Inport  Port=2
  ACCRequiredAccel : FVT_lib/inp/can_signal_template  SystemSampleTime=-1  VariantActivationTime=update diagram  Latency=0  AutoFrameSizeCalculation=off
      link override defval: Value=KINP_ACCRequiredAccel_mps2_defval
      link override fftdec: Value=KINP_ACCRequiredAccel_mps2_fftdec
      link override fftinc: Value=KINP_ACCRequiredAccel_mps2_fftinc
      link override fftlim: Value=KINP_ACCRequiredAccel_mps2_fftlim
      link override invalid: Value=KINP_ACCRequiredAccel_mps2_invalid
      link override ovrdflg: Value=KINP_ACCRequiredAccel_mps2_ovrdflg
      link override ovrdval: Value=KINP_ACCRequiredAccel_mps2_ovrdval
      link override setvalid: Value=KINP_ACCRequiredAccel_mps2_setvalid
      link override srvcflg: Value=KINP_ACCRequiredAccel_mps2_srvcflg
      link override srvcval: Value=KINP_ACCRequiredAccel_mps2_srvcval
  ACCVehHoldReq : FVT_lib/inp/can_signal_template  SystemSampleTime=-1  VariantActivationTime=update diagram  Latency=0  AutoFrameSizeCalculation=off
      link override defval: Value=KINP_ACCVehHoldReq_flg_defval
      link override fftdec: Value=KINP_ACCVehHoldReq_flg_fftdec
      link override fftinc: Value=KINP_ACCVehHoldReq_flg_fftinc
      link override fftlim: Value=KINP_ACCVehHoldReq_flg_fftlim
      link override invalid: Value=KINP_ACCVehHoldReq_flg_invalid
      link override ovrdflg: Value=KINP_ACCVehHoldReq_flg_ovrdflg
      link override ovrdval: Value=KINP_ACCVehHoldReq_flg_ovrdval
      link override setvalid: Value=KINP_ACCVehHoldReq_flg_setvalid
      link override srvcflg: Value=KINP_ACCVehHoldReq_flg_srvcflg
      link override srvcval: Value=KINP_ACCVehHoldReq_flg_srvcval
  FCM2CSErr : FVT_lib/inp/can_signal_template  SystemSampleTime=-1  VariantActivationTime=update diagram  Latency=0  AutoFrameSizeCalculation=off
      link override defval: Value=KINP_FCM2CSErr_flg_defval
      link override fftdec: Value=KINP_FCM2CSErr_flg_fftdec
      link override fftinc: Value=KINP_FCM2CSErr_flg_fftinc
      link override fftlim: Value=KINP_FCM2CSErr_flg_fftlim
      link override invalid: Value=KINP_FCM2CSErr_flg_invalid
      link override ovrdflg: Value=KINP_FCM2CSErr_flg_ovrdflg
      link override ovrdval: Value=KINP_FCM2CSErr_flg_ovrdval
      link override setvalid: Value=KINP_FCM2CSErr_flg_setvalid
      link override srvcflg: Value=KINP_FCM2CSErr_flg_srvcflg
      link override srvcval: Value=KINP_FCM2CSErr_flg_srvcval
  FCM2Checksum : FVT_lib/inp/can_signal_template  SystemSampleTime=-1  VariantActivationTime=update diagram  Latency=0  AutoFrameSizeCalculation=off
      link override defval: Value=KINP_FCM2Checksum_enum_defval
      link override fftdec: Value=KINP_FCM2Checksum_enum_fftdec
      link override fftinc: Value=KINP_FCM2Checksum_enum_fftinc
      link override fftlim: Value=KINP_FCM2Checksum_enum_fftlim
      link override invalid: Value=KINP_FCM2Checksum_enum_invalid
      link override ovrdflg: Value=KINP_FCM2Checksum_enum_ovrdflg
      link override ovrdval: Value=KINP_FCM2Checksum_enum_ovrdval
      link override setvalid: Value=KINP_FCM2Checksum_enum_setvalid
      link override srvcflg: Value=KINP_FCM2Checksum_enum_srvcflg
      link override srvcval: Value=KINP_FCM2Checksum_enum_srvcval
  FCM2LifeCount : FVT_lib/inp/can_signal_template  SystemSampleTime=-1  VariantActivationTime=update diagram  Latency=0  AutoFrameSizeCalculation=off
      link override defval: Value=KINP_FCM2LifeCount_enum_defval
      link override fftdec: Value=KINP_FCM2LifeCount_enum_fftdec
      link override fftinc: Value=KINP_FCM2LifeCount_enum_fftinc
      link override fftlim: Value=KINP_FCM2LifeCount_enum_fftlim
      link override invalid: Value=KINP_FCM2LifeCount_enum_invalid
      link override ovrdflg: Value=KINP_FCM2LifeCount_enum_ovrdflg
      link override ovrdval: Value=KINP_FCM2LifeCount_enum_ovrdval
      link override setvalid: Value=KINP_FCM2LifeCount_enum_setvalid
      link override srvcflg: Value=KINP_FCM2LifeCount_enum_srvcflg
      link override srvcval: Value=KINP_FCM2LifeCount_enum_srvcval
  FCM2RCErr : FVT_lib/inp/can_signal_template  SystemSampleTime=-1  VariantActivationTime=update diagram  Latency=0  AutoFrameSizeCalculation=off
      link override defval: Value=KINP_FCM2RCErr_flg_defval
      link override fftdec: Value=KINP_FCM2RCErr_flg_fftdec
      link override fftinc: Value=KINP_FCM2RCErr_flg_fftinc
      link override fftlim: Value=KINP_FCM2RCErr_flg_fftlim
      link override invalid: Value=KINP_FCM2RCErr_flg_invalid
      link override ovrdflg: Value=KINP_FCM2RCErr_flg_ovrdflg
      link override ovrdval: Value=KINP_FCM2RCErr_flg_ovrdval
      link override setvalid: Value=KINP_FCM2RCErr_flg_setvalid
      link override srvcflg: Value=KINP_FCM2RCErr_flg_srvcflg
      link override srvcval: Value=KINP_FCM2RCErr_flg_srvcval
  Terminator_{1..6} (6 alike) : Terminator
  True_VHAL_ACCRequiredAccel_mps2 : Constant  Value=TRUE  OutDataTypeStr=boolean
  True_VHAL_ACCVehHoldReq_flg : Constant  Value=TRUE  OutDataTypeStr=boolean
  True_VHAL_FCM2CSErr_flg : Constant  Value=TRUE  OutDataTypeStr=boolean
  True_VHAL_FCM2Checksum_enum : Constant  Value=TRUE  OutDataTypeStr=boolean
  True_VHAL_FCM2LifeCount_enum : Constant  Value=TRUE  OutDataTypeStr=boolean
  True_VHAL_FCM2RCErr_flg : Constant  Value=TRUE  OutDataTypeStr=boolean
  slr1_{1..6} (6 alike) : BusSelector  OutputSignals=VINP_CANMsgValidFCM2_flg
  slr_VHAL_ACCRequiredAccel_mps2 : BusSelector  OutputSignals=VHAL_ACCRequiredAccel_mps2
  slr_VHAL_ACCVehHoldReq_flg : BusSelector  OutputSignals=VHAL_ACCVehHoldReq_flg
  slr_VHAL_FCM2CSErr_flg : BusSelector  OutputSignals=VHAL_FCM2CSErr_flg
  slr_VHAL_FCM2Checksum_enum : BusSelector  OutputSignals=VHAL_FCM2Checksum_enum
  slr_VHAL_FCM2LifeCount_enum : BusSelector  OutputSignals=VHAL_FCM2LifeCount_enum
  slr_VHAL_FCM2RCErr_flg : BusSelector  OutputSignals=VHAL_FCM2RCErr_flg
  VINP_FCM2CSErr_flg : Outport
  VINP_FCM2RCErr_flg : Outport  Port=2
  VINP_ACCRequiredAccel_mps2 : Outport  Port=3
  VINP_ACCVehHoldReq_flg : Outport  Port=4
  VINP_FCM2Checksum_enum : Outport  Port=5
  VINP_FCM2LifeCount_enum : Outport  Port=6
  wires:
  BHAL_outputs/1 -> [BHAL_outputs]
  inp_CanValid_bus/1 -> [inp_CanValid_bus]
  [BHAL_outputs] -> slr_VHAL_FCM2CSErr_flg/1
  slr_VHAL_FCM2CSErr_flg/1 -> FCM2CSErr/1  "<VHAL_FCM2CSErr_flg>"
  True_VHAL_FCM2CSErr_flg/1 -> FCM2CSErr/2
  [inp_CanValid_bus] -> slr1_1/1
  slr1_1/1 -> FCM2CSErr/3  "<VINP_CANMsgValidFCM2_flg>"
  FCM2CSErr/1 -> VINP_FCM2CSErr_flg/1  "VINP_FCM2CSErr_flg"
  FCM2CSErr/2 -> Terminator_1/1
  [BHAL_outputs] -> slr_VHAL_FCM2RCErr_flg/1
  slr_VHAL_FCM2RCErr_flg/1 -> FCM2RCErr/1  "<VHAL_FCM2RCErr_flg>"
  True_VHAL_FCM2RCErr_flg/1 -> FCM2RCErr/2
  [inp_CanValid_bus] -> slr1_2/1
  slr1_2/1 -> FCM2RCErr/3  "<VINP_CANMsgValidFCM2_flg>"
  FCM2RCErr/1 -> VINP_FCM2RCErr_flg/1  "VINP_FCM2RCErr_flg"
  FCM2RCErr/2 -> Terminator_2/1
  [BHAL_outputs] -> slr_VHAL_ACCRequiredAccel_mps2/1
  slr_VHAL_ACCRequiredAccel_mps2/1 -> ACCRequiredAccel/1  "<VHAL_ACCRequiredAccel_mps2>"
  True_VHAL_ACCRequiredAccel_mps2/1 -> ACCRequiredAccel/2
  [inp_CanValid_bus] -> slr1_3/1
  slr1_3/1 -> ACCRequiredAccel/3  "<VINP_CANMsgValidFCM2_flg>"
  ACCRequiredAccel/1 -> VINP_ACCRequiredAccel_mps2/1  "VINP_ACCRequiredAccel_mps2"
  ACCRequiredAccel/2 -> Terminator_3/1
  [BHAL_outputs] -> slr_VHAL_ACCVehHoldReq_flg/1
  slr_VHAL_ACCVehHoldReq_flg/1 -> ACCVehHoldReq/1  "<VHAL_ACCVehHoldReq_flg>"
  True_VHAL_ACCVehHoldReq_flg/1 -> ACCVehHoldReq/2
  [inp_CanValid_bus] -> slr1_4/1
  slr1_4/1 -> ACCVehHoldReq/3  "<VINP_CANMsgValidFCM2_flg>"
  ACCVehHoldReq/1 -> VINP_ACCVehHoldReq_flg/1  "VINP_ACCVehHoldReq_flg"
  ACCVehHoldReq/2 -> Terminator_4/1
  [BHAL_outputs] -> slr_VHAL_FCM2Checksum_enum/1
  slr_VHAL_FCM2Checksum_enum/1 -> FCM2Checksum/1  "<VHAL_FCM2Checksum_enum>"
  True_VHAL_FCM2Checksum_enum/1 -> FCM2Checksum/2
  [inp_CanValid_bus] -> slr1_5/1
  slr1_5/1 -> FCM2Checksum/3  "<VINP_CANMsgValidFCM2_flg>"
  FCM2Checksum/1 -> VINP_FCM2Checksum_enum/1  "VINP_FCM2Checksum_enum"
  FCM2Checksum/2 -> Terminator_5/1
  [BHAL_outputs] -> slr_VHAL_FCM2LifeCount_enum/1
  slr_VHAL_FCM2LifeCount_enum/1 -> FCM2LifeCount/1  "<VHAL_FCM2LifeCount_enum>"
  True_VHAL_FCM2LifeCount_enum/1 -> FCM2LifeCount/2
  [inp_CanValid_bus] -> slr1_6/1
  slr1_6/1 -> FCM2LifeCount/3  "<VINP_CANMsgValidFCM2_flg>"
  FCM2LifeCount/1 -> VINP_FCM2LifeCount_enum/1  "VINP_FCM2LifeCount_enum"
  FCM2LifeCount/2 -> Terminator_6/1
